simulink model "different_terrains"  (Simulink 7.7)
settings: Solver=ode45  StartTime=0.0  StopTime=10  RelTol=1e-3
values from neighbouring files (symbols this model uses):
  b1 = 500    [initialise_parameters.m]
  b2 = 1500    [initialise_parameters.m]
  k1 = 60000*4    (= 240000)    [initialise_parameters.m]
  k2 = 1350000*4    (= 5400000)    [initialise_parameters.m]
  m1 = 500    [initialise_parameters.m]
  m2 = 50    [initialise_parameters.m]
undefined symbols (not defined in the file or in its folder): sigbuilder_block
libraries: simulink x3
settings Model: Creator=Rohan  LastModifiedBy=Rohan

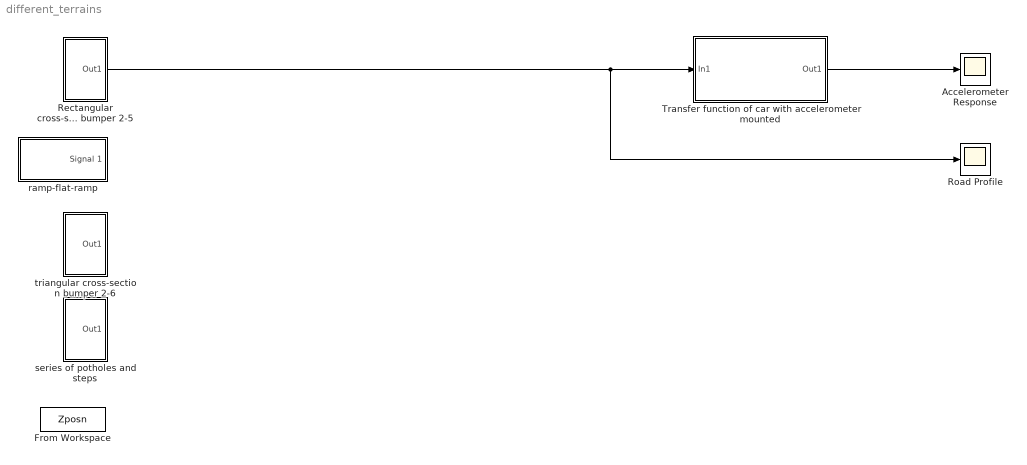
== system different_terrains ==
  Accelerometer Response : Scope
      settings: YMin=-90  YMax=25
  From Workspace : FromWorkspace  VariableName=Zposn  SampleTime=0
  Rectangular cross-section bumper 2-5 : Subsystem
  Road Profile : Scope
      settings: SaveName=ScopeData2
  Transfer function of car with accelerometer mounted : Subsystem
  ramp-flat-ramp : Subsystem  Tag=STV Subsys  LoadFcn=sigbuilder_block('load');  StartFcn=sigbuilder_block('start');  StopFcn=sigbuilder_block('stop');  ClipboardFcn=sigbuilder_block('clipboard');  mask(Sigbuilder block){}
      mask help: Create and generate interchangeable groups of signals whose waveforms are piecewise linear.
      mask init:
      | if ~strcmp(get_param(bdroot(gcbh),'SimulationStatus'),'stopped') tuvar = sigbuilder_block('maskInit'); end
      settings: CopyFcn=sigbuilder_block('copy');  DeleteFcn=sigbuilder_block('delete');  ModelCloseFcn=sigbuilder_block('modelClose');  PreSaveFcn=sigbuilder_block('preSave');  NameChangeFcn=sigbuilder_block('namechange');  OpenFcn=sigbuilder_block('open',[0 30 1024.5 489 ]);  CloseFcn=sigbuilder_block('close');
      mask Display: plot(0, 0, 100, 100,[2, 2, 32, 32, 2], [68, 8, 8, 68, 68],[32, 2], [38, 38], [32, 19, 2],[53, 60, 44], [32, 17, 17, 2],[16, 16, 31, 31]);txt = getActiveGroup(gcbh);text(2, 100, txt,'verticalAlignment', 'top');
  series of potholes and steps : Subsystem
  triangular cross-section bumper 2-6 : Subsystem
  wires:
  Transfer function of car with accelerometer mounted/1(Out1) -> Accelerometer Response/1
  Rectangular cross-section bumper 2-5/1(Out1) -> Transfer function of car with accelerometer mounted/1(In1), Road Profile/1

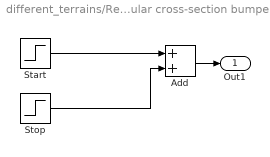
== system different_terrains/Rectangular cross-section bumper 2-5 ==
  Add : Sum
  Start : Step  Time=2  After=10  SampleTime=0
  Stop : Step  Time=5  After=-10  SampleTime=0
  Out1 : Outport
  wires:
  Stop/1 -> Add/2
  Start/1 -> Add/1
  Add/1 -> Out1/1

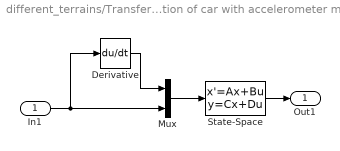
== system different_terrains/Transfer function of car with accelerometer mounted ==
  In1 : Inport
  Derivative : Derivative
  Mux : Mux  Inputs=2
  State-Space : StateSpace  A=[-b1/m1 b1/m1 -k1/m1 k1/m1; b1/m1 -(b1+b2)/m2 k1/m1 -(k1+k2)/m2;1 0 0 0; 0 1 0 0]  B=[0 0; b2/m2 k2/m2;0 0;0 0]  C=[0 0 1 0; 0 0 0 1; 0 0 1 -1]  D=[0 0;0 0;0 0]
  Out1 : Outport
  wires:
  Mux/1 -> State-Space/1
  Derivative/1 -> Mux/1
  In1/1 -> Derivative/1, Mux/2
  State-Space/1 -> Out1/1

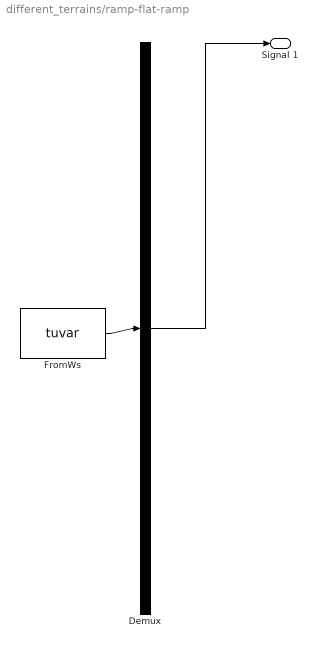
== system different_terrains/ramp-flat-ramp ==
  Demux : Demux  Tag=STV Demux  Outputs=1
  FromWs : FromWorkspace  Tag=STV FromWs  VariableName=tuvar  SampleTime=0  SigBuilderData=DataTag0  VnvData=DataTag1
      SigBuilderData=|
      | common.afterFinalStr = 'Extrapolate'
      | common.sampleTime = 0
      | dataSet.timeRange = [0 10]
      | dataSet.name = 'Group 1'
      | sbobj.Groups.Name = 'Group 1'
      | sbobj.Groups.Signals.Name = 'Signal 1'
      | sbobj.Groups.Signals.XData = [0 2 3 5 6 10]
      | sbobj.Groups.Signals.YData = [0 0 2 2 0 0]
  Signal 1 : Outport  Tag=STV Outport
  wires:
  Demux/1 -> Signal 1/1
  FromWs/1 -> Demux/1

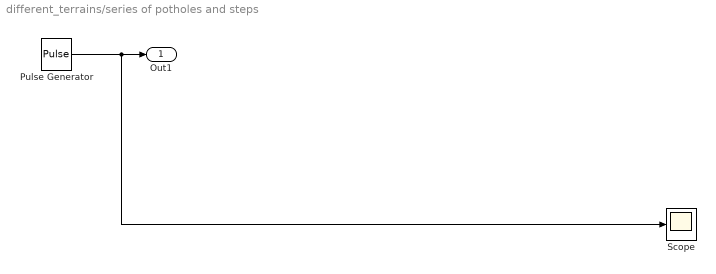
== system different_terrains/series of potholes and steps ==
  Pulse Generator : DiscretePulseGenerator  PulseType=Time based  Amplitude=5  Period=20  PulseWidth=50
  Scope : Scope
  Out1 : Outport
  wires:
  Pulse Generator/1 -> Out1/1, Scope/1

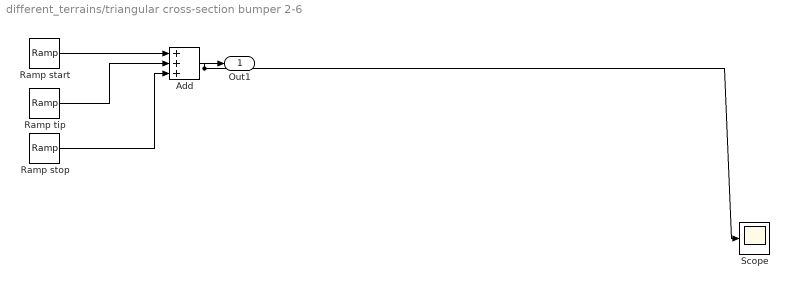
== system different_terrains/triangular cross-section bumper 2-6 ==
  Add : Sum  Inputs=+++
  Ramp start : simulink/Sources/Ramp  SystemSampleTime=-1  slope=1  start=2  X0=0
  Ramp stop : simulink/Sources/Ramp  SystemSampleTime=-1  slope=1  start=6  X0=0
  Ramp tip : simulink/Sources/Ramp  SystemSampleTime=-1  slope=-2  start=4  X0=0
  Scope : Scope
  Out1 : Outport
  wires:
  Ramp start/1 -> Add/1
  Add/1 -> Out1/1, Scope/1
  Ramp stop/1 -> Add/3
  Ramp tip/1 -> Add/2
